simulink model "RC_Response"  (R2023a)
settings: Solver=VariableStepAuto  StartTime=0.0  StopTime=3  RelTol=1e-3
settings Model: Creator=vselabs  LastModifiedBy=vselabs

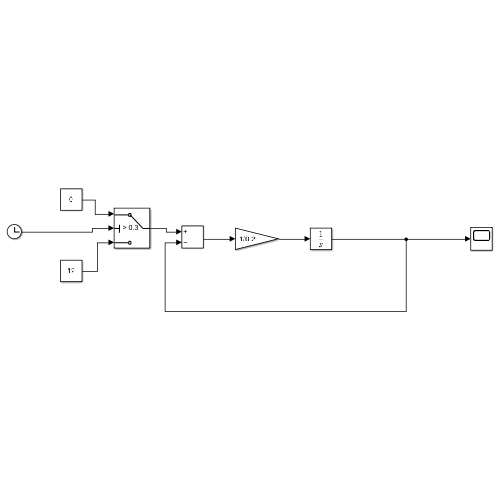
[thumbnail: Simulink's stored preview of the top-level diagram]
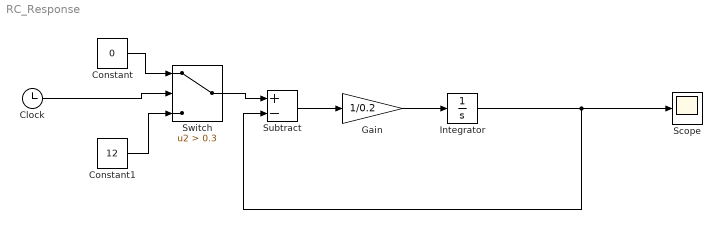
== system RC_Response ==
  Clock : Clock
  Constant : Constant  Value=0
  Constant1 : Constant  Value=12
  Gain : Gain  Gain=1/0.2
  Integrator : Integrator
  Scope : Scope
  Subtract : Sum  Inputs=+-
  Switch : Switch  Criteria=u2 > Threshold  Threshold=0.3  SaturateOnIntegerOverflow=off  InputSameDT=off
  wires:
  Integrator/1 -> Subtract/2, Scope/1
  Gain/1 -> Integrator/1
  Subtract/1 -> Gain/1
  Switch/1 -> Subtract/1
  Constant1/1 -> Switch/3
  Constant/1 -> Switch/1
  Clock/1 -> Switch/2
